simulink subsystem "EE_Dyn"  (R2022a)
settings: Solver=VariableStepAuto  StartTime=0.0  StopTime=10.0  RelTol=1e-3
model mask{spaceRobot=sr}
undefined symbols (not defined in the file): q_ddot
settings Model: Creator=charl  LastModifiedBy=charl

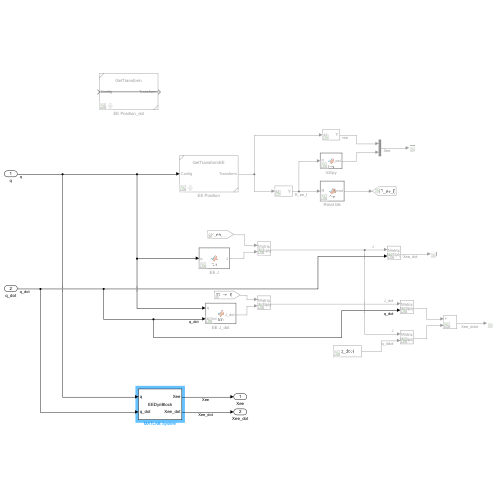
[thumbnail: Simulink's stored preview of the top-level diagram]
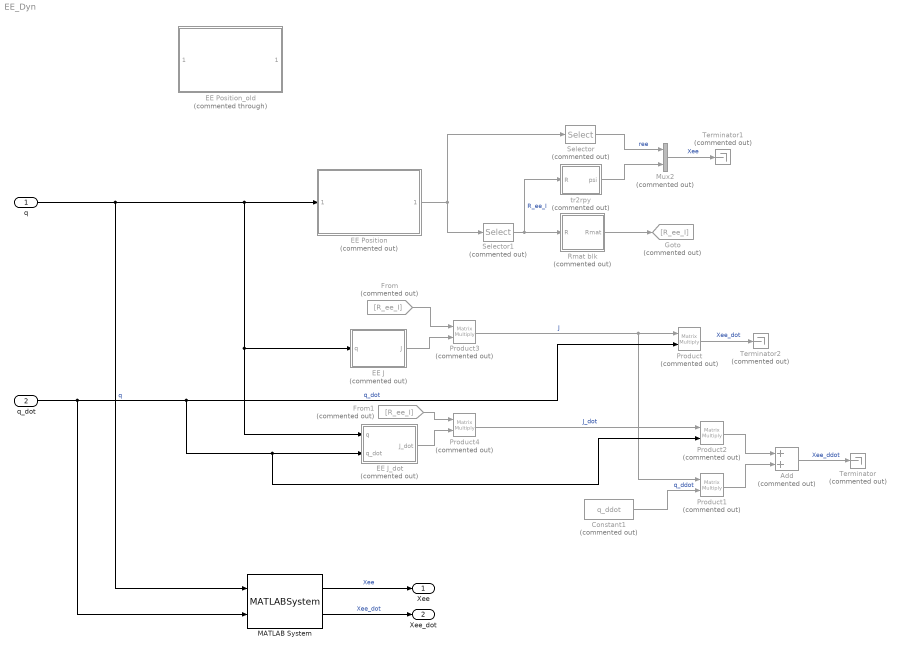
== system EE_Dyn ==
  q : Inport
  q_dot : Inport  Port=2
  Add : Sum  Commented=on
  Constant1 : Constant  Commented=on  Value=q_ddot
  EE J : MATLAB Function  Commented=on  TreatAsAtomicUnit=on
  EE J_dot : MATLAB Function  Commented=on  TreatAsAtomicUnit=on
  EE Position : Subsystem  Commented=on  ReferencedSubsystem=GetTransformEE  spaceRobot=sr
  EE Position_old : Subsystem  Commented=through  ReferencedSubsystem=GetTransform  spaceRobot=sr  sourceBody=endeffector  targetBody=inertial  SimulateUsing=Interpreted execution
  From : From  Commented=on  GotoTag=R_ee_I
  From1 : From  Commented=on  GotoTag=R_ee_I
  Goto : Goto  Commented=on  GotoTag=R_ee_I
  MATLAB System : MATLABSystem  System=EEDynBlock  srInfo=srInfo  srInfoFunc=srInfoFunc  srStateFunc=srStateFunc  srStateFuncMex=srStateFuncMex  SimulateUsing=Interpreted execution
      mask Type: EEDynBlock
      mask Display:
      | disp('EEDynBlock');
      | port_label('input',1,'q');
      | port_label('input',2,'q_dot');
      | port_label('output',1,'Xee');
      | port_label('output',2,'Xee_dot');
  Mux2 : Mux  Commented=on  Inputs=2
  Product{,1..4} (5 alike) : Product  Commented=on  Multiplication=Matrix(*)
  Rmat blk : MATLAB Function  Commented=on  TreatAsAtomicUnit=on
  Selector : Selector  Commented=on  NumberOfDimensions=2  InputPortWidth=[4 4]  IndexOptions=Index vector (dialog),Index vector (dialog)  Indices=[1:3],4  OutputSizes=1,1
  Selector1 : Selector  Commented=on  NumberOfDimensions=2  InputPortWidth=[4 4]  IndexOptions=Index vector (dialog),Index vector (dialog)  Indices=[1:3],[1:3]  OutputSizes=1,1
  Terminator : Terminator  Commented=on
  Terminator1 : Terminator  Commented=on
  Terminator2 : Terminator  Commented=on
  tr2rpy : MATLAB Function  Commented=on  TreatAsAtomicUnit=on
  Xee : Outport
  Xee_dot : Outport  Port=2
  wires:
  Selector1/1 -> Rmat blk/1(R), tr2rpy/1(R)  "R_ee_I"
  Product3/1 -> Product1/1, Product/1  "J"
  q_dot/1 -> EE J_dot/2(q_dot), Product2/2, Product/2, MATLAB System/2  "q_dot"
  EE J/1(J) -> Product3/2
  From/1 -> Product3/1
  Product2/1 -> Add/1
  EE Position/1 -> Selector1/1, Selector/1
  q/1 -> EE J_dot/1(q), EE J/1(q), EE Position/1, MATLAB System/1  "q"
  Product1/1 -> Add/2
  Selector/1 -> Mux2/1  "ree"
  Product4/1 -> Product2/1  "J_dot"
  Rmat blk/1(Rmat) -> Goto/1
  EE J_dot/1(J_dot) -> Product4/2
  Add/1 -> Terminator/1  "Xee_ddot"
  From1/1 -> Product4/1
  Constant1/1 -> Product1/2  "q_ddot"
  tr2rpy/1(psi) -> Mux2/2
  MATLAB System/1 -> Xee/1  "Xee"
  MATLAB System/2 -> Xee_dot/1  "Xee_dot"
  Mux2/1 -> Terminator1/1  "Xee"
  Product/1 -> Terminator2/1  "Xee_dot"

== matlab function EE_Dyn/EE J_dot ==
  data: q input; J_dot output; q_dot input
function J_dot = fcn(q, q_dot)
sr_info = SR2_info();

% 1 - Kinematics
[Rb, Ra, Rm] = RFunc_SR2(q);
Rm = reshape(Rm, 3, 3, []); % Split Rm to nk 3x3 arrays

% 2 - Kinetics
[t, ~, Omega, A, A_dot] = Kin(sr_info, q, q_dot, zeros(8, 1), {Rb, Ra, Rm});
wb = t{1}(4:6);

% 3 - J_dot
J_dot = Jacobian_dot('endeffector', sr_info, A, A_dot, {Rb, Ra}, wb, Omega);

== matlab function EE_Dyn/Rmat blk ==
  data: R input; Rmat output
function Rmat = fcn(R)

Rmat = blkdiag(R, R);

== matlab function EE_Dyn/tr2rpy ==
  data: R input; psi output size=[3, 1]
function psi = fcn(R)
% Computes euler angle from rotation matrix

psi = zeros(3, 1);

temp = rotm2eul(R, 'ZYX');
psi(1) = temp(3);
psi(2) = temp(2);
psi(3) = temp(1);

== matlab function EE_Dyn/EE J ==
  data: q input; J output; srInfoFunc parameter string
function J = fcn(q, srInfoFunc)

sr_info = feval(srInfoFunc);

% 1 - Kinematics
[Rb, Ra, Rm] = feval(sr_info.RFunc, q);
Rm = reshape(Rm, 3, 3, []); % Split Rm to nk 3x3 arrays

% 2 - Kinetics
[~, ~, ~, A, ~] = Kin(sr_info, q, zeros(sr_info.N, 1), zeros(sr_info.N, 1), {Rb, Ra, Rm});

% 3 - J
J = Jacobian('endeffector', sr_info, A, {Rb, Ra});

% J_dot = Jacobian_dot('endeffector', sr_info, A, A_dot, {Rb, Ra}, wb, Omega);

end
